simulink model "main_closed_loop"  (R2025b)
settings: Solver=FixedStepAuto  StartTime=0.0  StopTime=10.0  FixedStep=0.02  RelTol=1e-3
undefined symbols (not defined in the file or in its folder): Defined, driving, Ego, Lane, matlabshared, User
libraries: drivingscenarioandsensors x8, roadrunnerscenario x3, robotmobilelib x1, trackingutilitieslib x1, drivinglib x1
settings Model: Creator=Adarsh  LastModifiedBy=naman

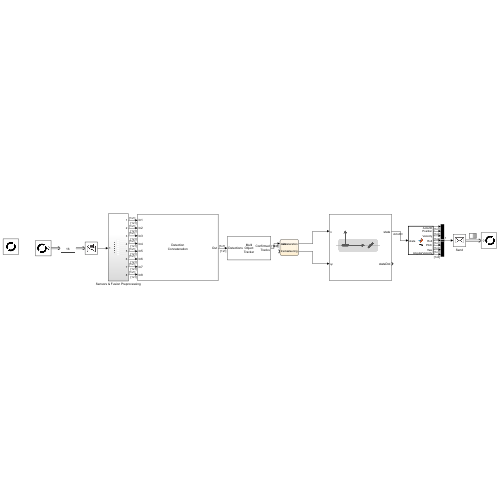
[thumbnail: Simulink's stored preview of the top-level diagram]
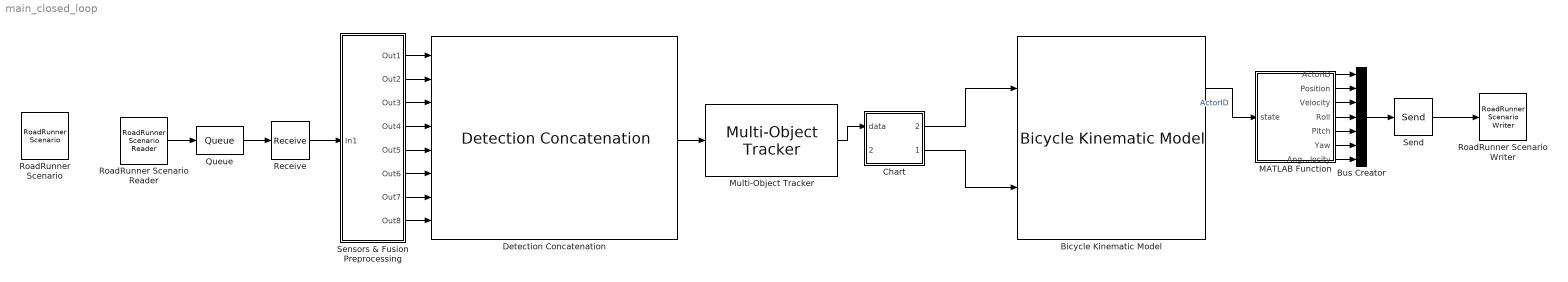
== system main_closed_loop ==
  Bicycle Kinematic Model : robotmobilelib/Bicycle Kinematic Model  VehicleInputs=Vehicle Speed & Steering Angle  WheelBase=1  VehicleSpeedRange=[-inf inf]  MaxSteeringAngle=pi/4  InitialState=[0; 0; 0]  SimulateUsing=Interpreted execution
  Bus Creator : BusCreator  Inputs=7  OutDataTypeStr=Bus: BusActorPose  NonVirtualBus=on
  Chart : Stateflow chart  TreatAsAtomicUnit=on
      settings: PortSchema="{\"entries\":[{\"content\":{\"sides\":[{\"content\":{\"connectorIds\":[\"In1\",\"In2\"]},\"type\":\"ConnectorPlacement.EquallySpacedRectSide\",\"uuid\":\"48cd63c9-5cf6-4ce7-a11d-983fc63462f6\"},{\"content\":{\"connectorIds\":[\"Out2\",\"Out1\"],\"side\":\"RIGHT\"},\"type\":\"ConnectorPlacement.EquallySpacedRectSide\",\"uuid\":\"b522bb60-53cf-4e9b-8133-3f4f00878f58\"},{\"content\":{\"side\":\"TOP\"},\"type\":\"ConnectorPlacement.EquallySpacedRectSide\",\"uuid\":\"8c295337-e204-4f24-a5e6-7f283fc49eb8\"}]},\"type\":\"ConnectorPlacement.EquallySpacedConnector\",\"uuid\":\"a3251784-4ce8-4ed7-8edd-8799e7b2b5f0\"}],\"packageUris\":[\"http://schema.mathworks.com/mf0/Connector/R2020b\"],\"version\":\"1.0\"}"
  Detection Concatenation : trackingutilitieslib/Detection Concatenation  NumInputs=8  BusNameSource=Auto  BusName=BusDetectionConcatenation  SimulateUsing=Interpreted execution
      settings: LibrarySourceBlock=drivinglib/Detection Concatenation
  MATLAB Function : MATLAB Function  TreatAsAtomicUnit=on
  Multi-Object Tracker : drivinglib/Multi-Object Tracker  TrackerIndex=uint32( 0 )  FilterInitializationFcn=initcvekf  AssignmentThreshold=30  ConfirmationThreshold=[4 5]  DeletionThreshold=[ 5, 5 ]  MaxNumTracks=20  MaxNumSensors=20  OOSMHandling=Terminate  StateParametersSimulink=struct  HasStateParametersInput=off  TimeInputSource=Auto  HasCostMatrixInput=off  HasDetectableTrackIDsInput=off  BusNameSource=Auto  BusName=BusMultiObjectTracker  TentativeTracksOutputPort=off  AllTracksOutputPort=off  SimulateUsing=Interpreted execution
  Queue : Queue  InputPortMessageModes=m  OutputPortMessageModes=m  OverwriteOldest=on  Capacity=16  QueueType=LIFO
  Receive : Receive  InputPortMessageModes=m  UseInternalQueue=off  QueueOverwriting=on  QueueLength=1  QueueType=LIFO
  RoadRunner Scenario : roadrunnerscenario/RoadRunner Scenario  UserDefinedActions={}  UserDefinedEvents={}  PathPoints=500
  RoadRunner Scenario Reader : roadrunnerscenario/RoadRunner Scenario Reader  TopicCategory=Actor  ActorCategory=All Types  ActionType=Path Following  EventType=User-Defined  TopicType=Actor Pose  VehicleType=Vehicle Specifications  TrafficSignalType=Traffic Signal Specifications  TrafficSignalControllerType=Traffic Signal Controller Specifications  UserDefinedAction=Action1  UserDefinedEvent=Event1  Filter=None  AdditionalRelationship=None  SensorTopic=Target Poses  LaneBoundaryOutputTopic=Ego-Lane  SensorID=1  SampleTime=0
  RoadRunner Scenario Writer : roadrunnerscenario/RoadRunner Scenario Writer  TopicCategory=Actor  ActorCategory=All Types  EventType=Action Complete  UserDefinedEvent=Event1  VehicleType=Vehicle Pose  TopicType=Actor Pose (Driving Scenario compatible)
  Send : Send  OutputPortMessageModes=m
  Sensors & Fusion Preprocessing : Subsystem
  wires:
  Detection Concatenation/1 -> Multi-Object Tracker/1
  Sensors & Fusion Preprocessing/1(Out1) -> Detection Concatenation/1
  Sensors & Fusion Preprocessing/2(Out2) -> Detection Concatenation/2
  Sensors & Fusion Preprocessing/3(Out3) -> Detection Concatenation/3
  Sensors & Fusion Preprocessing/4(Out4) -> Detection Concatenation/4
  Sensors & Fusion Preprocessing/5(Out5) -> Detection Concatenation/5
  Sensors & Fusion Preprocessing/6(Out6) -> Detection Concatenation/6
  Sensors & Fusion Preprocessing/7(Out7) -> Detection Concatenation/7
  Sensors & Fusion Preprocessing/8(Out8) -> Detection Concatenation/8
  Multi-Object Tracker/1 -> Chart/1(data)
  Chart/2(acceleration) -> Bicycle Kinematic Model/1
  Chart/1(steering) -> Bicycle Kinematic Model/2
  RoadRunner Scenario Reader/1 -> Queue/1
  Queue/1 -> Receive/1
  Receive/1 -> Sensors & Fusion Preprocessing/1(In1)
  Bicycle Kinematic Model/1 -> MATLAB Function/1(state)  "ActorID"
  Send/1 -> RoadRunner Scenario Writer/1
  MATLAB Function/1(ActorID) -> Bus Creator/1
  MATLAB Function/2(Position) -> Bus Creator/2
  MATLAB Function/3(Velocity) -> Bus Creator/3
  MATLAB Function/4(Roll) -> Bus Creator/4
  Bus Creator/1 -> Send/1
  MATLAB Function/5(Pitch) -> Bus Creator/5
  MATLAB Function/6(Yaw) -> Bus Creator/6
  MATLAB Function/7(AngularVelocity) -> Bus Creator/7

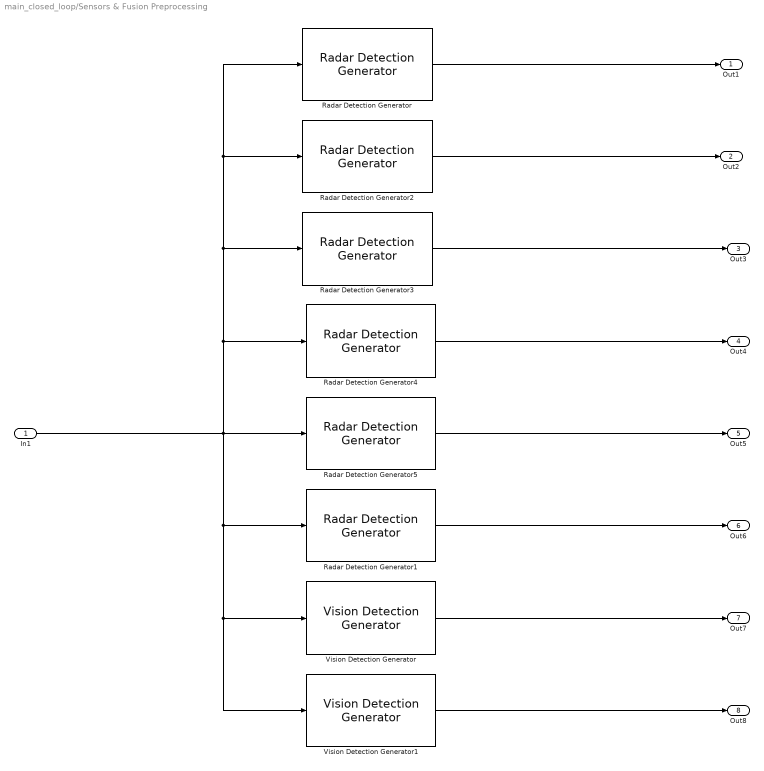
== system main_closed_loop/Sensors & Fusion Preprocessing ==
  In1 : Inport
  Radar Detection Generator : drivingscenarioandsensors/Radar Detection Generator  SensorIndex=1  UpdateInterval=0.1  SensorLocation=[ 3.4, 0 ]  Height=0.2  Yaw=0  Pitch=0  Roll=0  BusNameSource=Auto  BusName=BusRadarDetectionGenerator  MaxNumDetectionsSource=Property  MaxNumDetections=50  DetectionCoordinates=Ego Cartesian  SimulateUsing=Interpreted execution  AzimuthResolution=4  ElevationResolution=10  RangeResolution=2.5  RangeRateResolution=0.5  AzimuthBiasFraction=0.1  ElevationBiasFraction=0.1  RangeBiasFraction=0.05  RangeRateBiasFraction=0.05  FieldOfView=[ 20, 5 ]  MaxRange=150  RangeRateLimits=[ -100, 100 ]  DetectionProbability=0.9  FalseAlarmRate=1e-6  ReferenceRange=100  ReferenceRCS=0  HasElevation=off  HasRangeRate=on  HasNoise=on  HasFalseAlarms=on  HasOcclusion=on  InitialSeedSource=Repeatable  InitialSeed=0  UsedSeed=matlabshared.tracking.internal.SimulinkUtilities.seedManager(gcb)  ActorProfilesSource=Parameters  ActorProfilesParameters=driving.internal.ActorProfilesRadarParameters  ActorProfilesExpression=struct( 'ClassID', 0, 'Length', 4.7, 'Width', 1.8, 'Height', 1.4, 'OriginOffset', [ -1.35, 0, 0 ], 'RCSPattern', [ 10, 10; 10, 10 ], 'RCSAzimuthAngles', [ -180, 180 ], 'RCSElevationAngles', [ -90, 90 ] )
  Radar Detection Generator1 : drivingscenarioandsensors/Radar Detection Generator  SensorIndex=6  UpdateInterval=0.1  SensorLocation=[ 3.4, 0 ]  Height=0.2  Yaw=0  Pitch=0  Roll=0  BusNameSource=Auto  BusName=BusRadarDetectionGenerator  MaxNumDetectionsSource=Property  MaxNumDetections=50  DetectionCoordinates=Ego Cartesian  SimulateUsing=Interpreted execution  AzimuthResolution=4  ElevationResolution=10  RangeResolution=2.5  RangeRateResolution=0.5  AzimuthBiasFraction=0.1  ElevationBiasFraction=0.1  RangeBiasFraction=0.05  RangeRateBiasFraction=0.05  FieldOfView=[ 20, 5 ]  MaxRange=150  RangeRateLimits=[ -100, 100 ]  DetectionProbability=0.9  FalseAlarmRate=1e-6  ReferenceRange=100  ReferenceRCS=0  HasElevation=off  HasRangeRate=on  HasNoise=on  HasFalseAlarms=on  HasOcclusion=on  InitialSeedSource=Repeatable  InitialSeed=0  UsedSeed=matlabshared.tracking.internal.SimulinkUtilities.seedManager(gcb)  ActorProfilesSource=Parameters  ActorProfilesParameters=driving.internal.ActorProfilesRadarParameters  ActorProfilesExpression=struct( 'ClassID', 0, 'Length', 4.7, 'Width', 1.8, 'Height', 1.4, 'OriginOffset', [ -1.35, 0, 0 ], 'RCSPattern', [ 10, 10; 10, 10 ], 'RCSAzimuthAngles', [ -180, 180 ], 'RCSElevationAngles', [ -90, 90 ] )
  Radar Detection Generator2 : drivingscenarioandsensors/Radar Detection Generator  SensorIndex=2  UpdateInterval=0.1  SensorLocation=[ 3.4, 0 ]  Height=0.2  Yaw=0  Pitch=0  Roll=0  BusNameSource=Auto  BusName=BusRadarDetectionGenerator  MaxNumDetectionsSource=Property  MaxNumDetections=50  DetectionCoordinates=Ego Cartesian  SimulateUsing=Interpreted execution  AzimuthResolution=4  ElevationResolution=10  RangeResolution=2.5  RangeRateResolution=0.5  AzimuthBiasFraction=0.1  ElevationBiasFraction=0.1  RangeBiasFraction=0.05  RangeRateBiasFraction=0.05  FieldOfView=[ 20, 5 ]  MaxRange=150  RangeRateLimits=[ -100, 100 ]  DetectionProbability=0.9  FalseAlarmRate=1e-6  ReferenceRange=100  ReferenceRCS=0  HasElevation=off  HasRangeRate=on  HasNoise=on  HasFalseAlarms=on  HasOcclusion=on  InitialSeedSource=Repeatable  InitialSeed=0  UsedSeed=matlabshared.tracking.internal.SimulinkUtilities.seedManager(gcb)  ActorProfilesSource=Parameters  ActorProfilesParameters=driving.internal.ActorProfilesRadarParameters  ActorProfilesExpression=struct( 'ClassID', 0, 'Length', 4.7, 'Width', 1.8, 'Height', 1.4, 'OriginOffset', [ -1.35, 0, 0 ], 'RCSPattern', [ 10, 10; 10, 10 ], 'RCSAzimuthAngles', [ -180, 180 ], 'RCSElevationAngles', [ -90, 90 ] )
  Radar Detection Generator3 : drivingscenarioandsensors/Radar Detection Generator  SensorIndex=3  UpdateInterval=0.1  SensorLocation=[ 3.4, 0 ]  Height=0.2  Yaw=0  Pitch=0  Roll=0  BusNameSource=Auto  BusName=BusRadarDetectionGenerator  MaxNumDetectionsSource=Property  MaxNumDetections=50  DetectionCoordinates=Ego Cartesian  SimulateUsing=Interpreted execution  AzimuthResolution=4  ElevationResolution=10  RangeResolution=2.5  RangeRateResolution=0.5  AzimuthBiasFraction=0.1  ElevationBiasFraction=0.1  RangeBiasFraction=0.05  RangeRateBiasFraction=0.05  FieldOfView=[ 20, 5 ]  MaxRange=150  RangeRateLimits=[ -100, 100 ]  DetectionProbability=0.9  FalseAlarmRate=1e-6  ReferenceRange=100  ReferenceRCS=0  HasElevation=off  HasRangeRate=on  HasNoise=on  HasFalseAlarms=on  HasOcclusion=on  InitialSeedSource=Repeatable  InitialSeed=0  UsedSeed=matlabshared.tracking.internal.SimulinkUtilities.seedManager(gcb)  ActorProfilesSource=Parameters  ActorProfilesParameters=driving.internal.ActorProfilesRadarParameters  ActorProfilesExpression=struct( 'ClassID', 0, 'Length', 4.7, 'Width', 1.8, 'Height', 1.4, 'OriginOffset', [ -1.35, 0, 0 ], 'RCSPattern', [ 10, 10; 10, 10 ], 'RCSAzimuthAngles', [ -180, 180 ], 'RCSElevationAngles', [ -90, 90 ] )
  Radar Detection Generator4 : drivingscenarioandsensors/Radar Detection Generator  SensorIndex=4  UpdateInterval=0.1  SensorLocation=[ 3.4, 0 ]  Height=0.2  Yaw=0  Pitch=0  Roll=0  BusNameSource=Auto  BusName=BusRadarDetectionGenerator  MaxNumDetectionsSource=Property  MaxNumDetections=50  DetectionCoordinates=Ego Cartesian  SimulateUsing=Interpreted execution  AzimuthResolution=4  ElevationResolution=10  RangeResolution=2.5  RangeRateResolution=0.5  AzimuthBiasFraction=0.1  ElevationBiasFraction=0.1  RangeBiasFraction=0.05  RangeRateBiasFraction=0.05  FieldOfView=[ 20, 5 ]  MaxRange=150  RangeRateLimits=[ -100, 100 ]  DetectionProbability=0.9  FalseAlarmRate=1e-6  ReferenceRange=100  ReferenceRCS=0  HasElevation=off  HasRangeRate=on  HasNoise=on  HasFalseAlarms=on  HasOcclusion=on  InitialSeedSource=Repeatable  InitialSeed=0  UsedSeed=matlabshared.tracking.internal.SimulinkUtilities.seedManager(gcb)  ActorProfilesSource=Parameters  ActorProfilesParameters=driving.internal.ActorProfilesRadarParameters  ActorProfilesExpression=struct( 'ClassID', 0, 'Length', 4.7, 'Width', 1.8, 'Height', 1.4, 'OriginOffset', [ -1.35, 0, 0 ], 'RCSPattern', [ 10, 10; 10, 10 ], 'RCSAzimuthAngles', [ -180, 180 ], 'RCSElevationAngles', [ -90, 90 ] )
  Radar Detection Generator5 : drivingscenarioandsensors/Radar Detection Generator  SensorIndex=5  UpdateInterval=0.1  SensorLocation=[ 3.4, 0 ]  Height=0.2  Yaw=0  Pitch=0  Roll=0  BusNameSource=Auto  BusName=BusRadarDetectionGenerator  MaxNumDetectionsSource=Property  MaxNumDetections=50  DetectionCoordinates=Ego Cartesian  SimulateUsing=Interpreted execution  AzimuthResolution=4  ElevationResolution=10  RangeResolution=2.5  RangeRateResolution=0.5  AzimuthBiasFraction=0.1  ElevationBiasFraction=0.1  RangeBiasFraction=0.05  RangeRateBiasFraction=0.05  FieldOfView=[ 20, 5 ]  MaxRange=150  RangeRateLimits=[ -100, 100 ]  DetectionProbability=0.9  FalseAlarmRate=1e-6  ReferenceRange=100  ReferenceRCS=0  HasElevation=off  HasRangeRate=on  HasNoise=on  HasFalseAlarms=on  HasOcclusion=on  InitialSeedSource=Repeatable  InitialSeed=0  UsedSeed=matlabshared.tracking.internal.SimulinkUtilities.seedManager(gcb)  ActorProfilesSource=Parameters  ActorProfilesParameters=driving.internal.ActorProfilesRadarParameters  ActorProfilesExpression=struct( 'ClassID', 0, 'Length', 4.7, 'Width', 1.8, 'Height', 1.4, 'OriginOffset', [ -1.35, 0, 0 ], 'RCSPattern', [ 10, 10; 10, 10 ], 'RCSAzimuthAngles', [ -180, 180 ], 'RCSElevationAngles', [ -90, 90 ] )
  Vision Detection Generator : drivingscenarioandsensors/Vision Detection Generator  SensorIndex=7  DetectorOutput=Objects only  UpdateInterval=0.1  LaneUpdateInterval=0.1  SensorLocation=[ 1.9, 0 ]  Height=1.1  Yaw=0  Pitch=1  Roll=0  BusNameSource=Auto  BusName=BusObjectDetections  BusName2Source=Auto  BusName2=BusLaneDetections  MaxNumDetectionsSource=Property  MaxNumDetections=50  MaxNumLanesSource=Property  MaxNumLanes=30  DetectionCoordinates=Ego Cartesian  SimulateUsing=Interpreted execution  MaxRange=150  BoundingBoxAccuracy=5  ProcessNoiseIntensity=5  MaxSpeed=100  MaxAllowedOcclusion=0.5  MinObjectImageSize=[ 15, 15 ]  DetectionProbability=0.9  FalsePositivesPerImage=0.1  MinLaneImageSize=[ 20, 3 ]  LaneBoundaryAccuracy=3  HasNoise=on  InitialSeedSource=Repeatable  InitialSeed=0  UsedSeed=driving.internal.SimulinkUtilities.seedManager(gcb)  ActorProfilesSource=From Scenario Reader block  ActorProfilesParameters=driving.internal.ActorProfilesParameters  ActorProfilesExpression=struct( 'ClassID', 0, 'Length', 4.7, 'Width', 1.8, 'Height', 1.4, 'OriginOffset', [ -1.35, 0, 0 ] )  Intrinsics=driving.internal.cameraIntrinsics
  Vision Detection Generator1 : drivingscenarioandsensors/Vision Detection Generator  SensorIndex=8  DetectorOutput=Objects only  UpdateInterval=0.1  LaneUpdateInterval=0.1  SensorLocation=[ 1.9, 0 ]  Height=1.1  Yaw=0  Pitch=1  Roll=0  BusNameSource=Auto  BusName=BusObjectDetections  BusName2Source=Auto  BusName2=BusLaneDetections  MaxNumDetectionsSource=Property  MaxNumDetections=50  MaxNumLanesSource=Property  MaxNumLanes=30  DetectionCoordinates=Ego Cartesian  SimulateUsing=Interpreted execution  MaxRange=150  BoundingBoxAccuracy=5  ProcessNoiseIntensity=5  MaxSpeed=100  MaxAllowedOcclusion=0.5  MinObjectImageSize=[ 15, 15 ]  DetectionProbability=0.9  FalsePositivesPerImage=0.1  MinLaneImageSize=[ 20, 3 ]  LaneBoundaryAccuracy=3  HasNoise=on  InitialSeedSource=Repeatable  InitialSeed=0  UsedSeed=driving.internal.SimulinkUtilities.seedManager(gcb)  ActorProfilesSource=From Scenario Reader block  ActorProfilesParameters=driving.internal.ActorProfilesParameters  ActorProfilesExpression=struct( 'ClassID', 0, 'Length', 4.7, 'Width', 1.8, 'Height', 1.4, 'OriginOffset', [ -1.35, 0, 0 ] )  Intrinsics=driving.internal.cameraIntrinsics
  Out1 : Outport
  Out2 : Outport  Port=2
  Out3 : Outport  Port=3
  Out4 : Outport  Port=4
  Out5 : Outport  Port=5
  Out6 : Outport  Port=6
  Out7 : Outport  Port=7
  Out8 : Outport  Port=8
  wires:
  Radar Detection Generator4/1 -> Out4/1
  Vision Detection Generator/1 -> Out7/1
  Radar Detection Generator1/1 -> Out6/1
  Vision Detection Generator1/1 -> Out8/1
  Radar Detection Generator5/1 -> Out5/1
  Radar Detection Generator3/1 -> Out3/1
  Radar Detection Generator2/1 -> Out2/1
  In1/1 -> Vision Detection Generator1/1, Vision Detection Generator/1, Radar Detection Generator1/1, Radar Detection Generator/1, Radar Detection Generator2/1, Radar Detection Generator3/1, Radar Detection Generator4/1, Radar Detection Generator5/1
  Radar Detection Generator/1 -> Out1/1

== matlab function main_closed_loop/MATLAB Function ==
  data: state input; ActorID output; Position output; Velocity output; Roll output; Pitch output; Yaw output; AngularVelocity output
function [ActorID, Position, Velocity, Roll, Pitch, Yaw, AngularVelocity] = fcn(state)
% Unpack 2D kinematic state [x, y, psi, v]
x   = double(state(1));
y   = double(state(2));
psi = double(state(3));   % radians
v   = double(state(4));

ActorID         = double(1);
Position        = [x, y, 0];
Velocity        = [v*cos(psi), v*sin(psi), 0];
Roll            = double(0);
Pitch           = double(0);
Yaw             = psi * 180/pi;     % BusActorPose expects degrees, not radians
AngularVelocity = [0, 0, 0];
end

== stateflow chart main_closed_loop/Chart ==
  state NominalDriving
    during:
    % Default behavior (nominal driving)
    steering = 0.0;
    acceleration = 2.0;
    % Check if any tracked obstacles exist
    if ~isempty(tracks)
    for i = 1:length(tracks)
    % tracks(i).State(1) is longitudinal distance (X)
    % tracks(i).State(3) is lateral distance (Y)
    xDist = tracks(i).State(1);
    yDist = tracks(i).State(3);
    % If an obstacle is ahead (0 to 20 meters) and in your lane (+/- 1.5m)
    if xDist > 0 && xDist < 20 && abs(yDist) < 1.5
    acceleration = -4.0; % Apply braking
    steering = 0.3;      % Swerve away
    end
    end
    end
  (default) -> NominalDriving
  data: data input; steering output; acceleration output; tracks input size=[1 20]; i local; xDist local; yDist local
